simulink model "EF20Algo"  (R2020a)
settings: Solver=VariableStepAuto  StartTime=0.0  StopTime=10.0  RelTol=1e-3
model workspace (MAT data in the model file):
  Batt.init_charge = 100
  Batt.Vnom = 320
  Batt.Ah_rating = 100
  Batt.R1 = 0.0846
  Batt.V1 = 283.3
  Batt.Q1 = 10.4
  Batt.Limit.SOC = [0 10 20 30 40 50 60 70 80 90 100]
  Batt.Limit.Discharge = [0 15000 33000 54000 75000 90000 108000 117000 120000 120000 120000]
  Batt.Limit.Charge = [1 1 1 1 1 1 1 1 0.75 0.35 0]
  Batt.m = 119.7
  Batt.Cp = 101.079756
undefined symbols (not defined in the file): magnitude
libraries: simulink x4
settings Model: Creator=Administrator  LastModifiedBy=Administrator

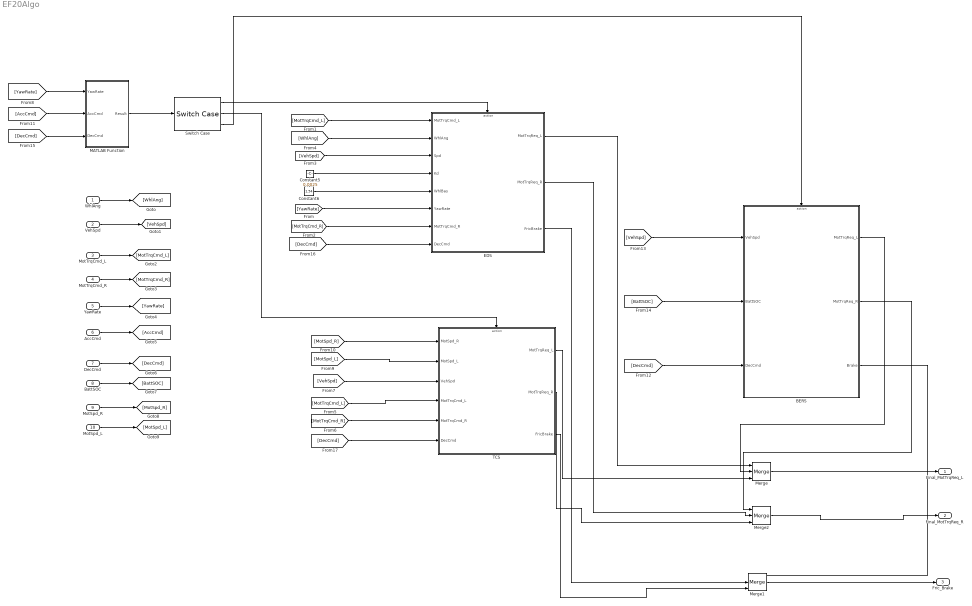
== system EF20Algo ==
  WhlAng : Inport
  VehSpd : Inport  Port=2
  MotTrqCmd_L : Inport  Port=3
  MotTrqCmd_R : Inport  Port=4
  YawRate : Inport  Port=5
  AccCmd : Inport  Port=6
  DecCmd : Inport  Port=7
  BattSOC : Inport  Port=8
  MotSpd_R : Inport  Port=9
  MotSpd_L : Inport  Port=10
  BERS : Subsystem  TreatAsAtomicUnit=on
  Constant5 : Constant  Value=0.0025
  Constant6 : Constant  Value=1.54
  EDS : Subsystem  TreatAsAtomicUnit=on
  MATLAB Function : MATLAB Function  TreatAsAtomicUnit=on
  Merge : Merge  Inputs=3
  Merge1 : Merge  Inputs=3
  Merge2 : Merge  Inputs=3
  Switch Case : SwitchCase  CaseConditions={1,2,3}  ShowDefaultCase=off
  TCS : Subsystem  TreatAsAtomicUnit=on
  Final_MotTrqReq_L : Outport
  Final_MotTrqReq_R : Outport  Port=2
  Fric_Brake : Outport  Port=3
  wires:
  WhlAng/1 -> [WhlAng]
  MotSpd_R/1 -> [MotSpd_R]
  DecCmd/1 -> [DecCmd]
  BattSOC/1 -> [BattSOC]
  MotSpd_L/1 -> [MotSpd_L]
  AccCmd/1 -> [AccCmd]
  YawRate/1 -> [YawRate]
  MotTrqCmd_R/1 -> [MotTrqCmd_R]
  MotTrqCmd_L/1 -> [MotTrqCmd_L]
  VehSpd/1 -> [VehSpd]
  Switch Case/2 -> TCS/Action
  Switch Case/1 -> EDS/Action
  Constant5/1 -> EDS/4(Kd)
  Constant6/1 -> EDS/5(WhlBas)
  [YawRate] -> EDS/6(YawRate)
  [MotTrqCmd_L] -> EDS/1(MotTrqCmd_L)
  [MotTrqCmd_R] -> EDS/7(MotTrqCmd_R)
  [WhlAng] -> EDS/2(WhlAng)
  [VehSpd] -> EDS/3(Spd)
  [MotSpd_L] -> TCS/2(MotSpd_L)
  [MotSpd_R] -> TCS/1(MotSpd_R)
  [VehSpd] -> TCS/3(VehSpd)
  [MotTrqCmd_L] -> TCS/4(MotTrqCmd_L)
  [MotTrqCmd_R] -> TCS/5(MotTrqCmd_R)
  MATLAB Function/1(Result) -> Switch Case/1
  [YawRate] -> MATLAB Function/1(YawRate)
  [AccCmd] -> MATLAB Function/2(AccCmd)
  [VehSpd] -> BERS/1(VehSpd)
  [BattSOC] -> BERS/2(BattSOC)
  [DecCmd] -> BERS/3(DecCmd)
  [DecCmd] -> MATLAB Function/3(DecCmd)
  Switch Case/3 -> BERS/Action
  [DecCmd] -> EDS/8(DecCmd)
  [DecCmd] -> TCS/6(DecCmd)
  Merge1/1 -> Fric_Brake/1
  Merge2/1 -> Final_MotTrqReq_R/1
  Merge/1 -> Final_MotTrqReq_L/1
  EDS/1(MotTrqReq_L) -> Merge/1
  BERS/1(MotTrqReq_L) -> Merge/2
  TCS/1(MotTrqReq_L) -> Merge/3
  BERS/2(MotTrqReq_R) -> Merge2/1
  EDS/2(MotTrqReq_R) -> Merge2/2
  TCS/2(MotTrqReq_R) -> Merge2/3
  BERS/3(Brake) -> Merge1/1
  EDS/3(FricBrake) -> Merge1/2
  TCS/3(FricBrake) -> Merge1/3

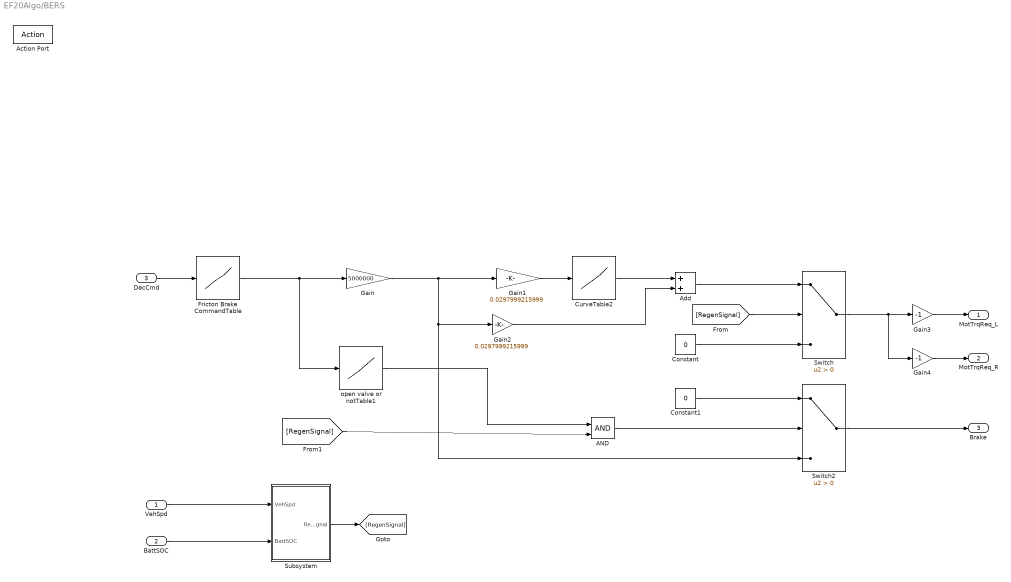
== system EF20Algo/BERS ==
  VehSpd : Inport
  BattSOC : Inport  Port=2
  DecCmd : Inport  Port=3
  Action Port : ActionPort  ActionPortLabel=case [ 3 ]:
  AND : Logic  IconShape=distinctive  AllPortsSameDT=off  OutDataTypeStr=boolean
  Add : Sum
  Constant : Constant  Value=0
  Constant1 : Constant  Value=0
  CurveTable2 : Lookup_n-D  NumberOfTableDimensions=1  BreakpointsForDimension1=Batt.Limit.SOC  Table=Batt.Limit.Charge  InternalRulePriority=Speed  RndMeth=Simplest  InputSameDT=on
  Fricton Brake CommandTable : Lookup_n-D  NumberOfTableDimensions=1  BreakpointsForDimension1=[.0 0.1 0.2 0.4 0.6 0.8 1.0]  Table=[0 0 0.2 0.4 0.6 0.8 1.0]*60  InternalRulePriority=Speed  RndMeth=Simplest  InputSameDT=on
  Gain : Gain  Gain=5000000
  Gain1 : Gain  Gain=0.0297999215999
  Gain2 : Gain  Gain=0.0297999215999
  Gain3 : Gain  Gain=-1
  Gain4 : Gain  Gain=-1
  Subsystem : Subsystem
  Switch : Switch  Criteria=u2 > Threshold
  Switch2 : Switch  Criteria=u2 > Threshold
  open valve or notTable1 : Lookup_n-D  NumberOfTableDimensions=1  BreakpointsForDimension1=[.0 0.1 0.2 0.4 0.6 0.8 1.0]  Table=[0 0 0.2 0.4 0.6 0.8 1.0]*60  InternalRulePriority=Speed  RndMeth=Simplest  InputSameDT=on
  MotTrqReq_L : Outport
  MotTrqReq_R : Outport  Port=2
  Brake : Outport  Port=3
  wires:
  Fricton Brake CommandTable/1 -> open valve or notTable1/1, Gain/1
  Subsystem/1(RegenSignal) -> [RegenSignal]
  Gain3/1 -> MotTrqReq_L/1
  [RegenSignal] -> AND/2
  BattSOC/1 -> Subsystem/2(BattSOC)
  Gain4/1 -> MotTrqReq_R/1
  Gain2/1 -> Add/2
  Switch/1 -> Gain4/1, Gain3/1
  Switch2/1 -> Brake/1
  Gain1/1 -> CurveTable2/1
  CurveTable2/1 -> Add/1
  [RegenSignal] -> Switch/2
  Gain/1 -> Switch2/3, Gain2/1, Gain1/1
  Constant/1 -> Switch/3
  Constant1/1 -> Switch2/1
  VehSpd/1 -> Subsystem/1(VehSpd)
  open valve or notTable1/1 -> AND/1
  Add/1 -> Switch/1
  AND/1 -> Switch2/2
  DecCmd/1 -> Fricton Brake CommandTable/1

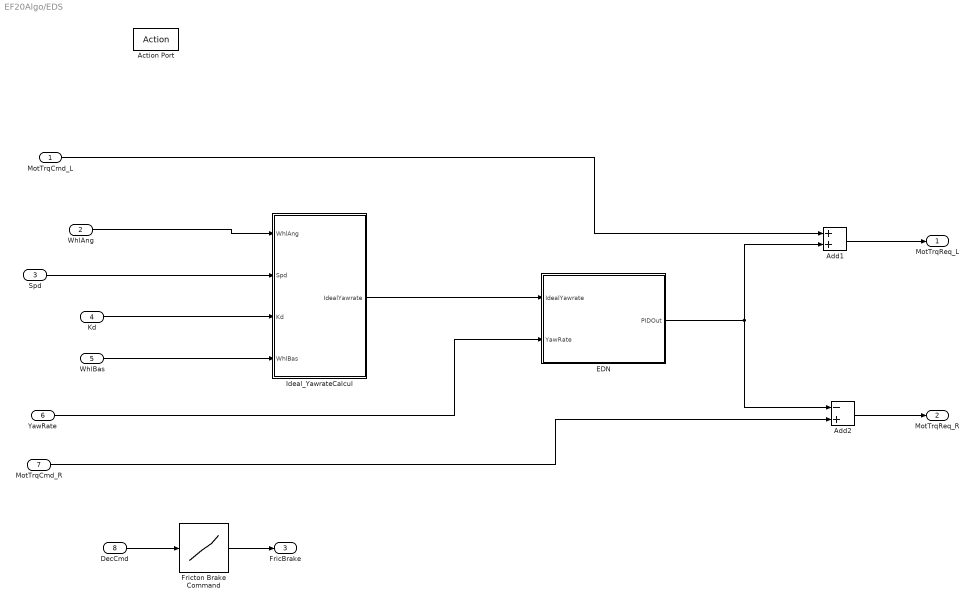
== system EF20Algo/EDS ==
  MotTrqCmd_L : Inport
  WhlAng : Inport  Port=2
  Spd : Inport  Port=3
  Kd : Inport  Port=4
  WhlBas : Inport  Port=5
  YawRate : Inport  Port=6
  MotTrqCmd_R : Inport  Port=7
  DecCmd : Inport  Port=8
  Action Port : ActionPort  ActionPortLabel=case [ 1 ]:
  Add1 : Sum
  Add2 : Sum  Inputs=-+
  EDN : Subsystem
  Fricton Brake Command : Lookup_n-D  NumberOfTableDimensions=1  BreakpointsForDimension1=[.0 0.1 0.2 0.4 0.6 0.8 1.0]  Table=[0 0 0.2 0.4 0.6 0.8 1.0]*60  ExtrapMethod=Clip  InternalRulePriority=Speed  RndMeth=Simplest  InputSameDT=on
  Ideal_YawrateCalcul : Subsystem
  MotTrqReq_L : Outport
  MotTrqReq_R : Outport  Port=2
  FricBrake : Outport  Port=3
  wires:
  Ideal_YawrateCalcul/1(IdealYawrate) -> EDN/1(IdealYawrate)
  Add2/1 -> MotTrqReq_R/1
  Add1/1 -> MotTrqReq_L/1
  YawRate/1 -> EDN/2(YawRate)
  Spd/1 -> Ideal_YawrateCalcul/2(Spd)
  MotTrqCmd_L/1 -> Add1/1
  WhlBas/1 -> Ideal_YawrateCalcul/4(WhlBas)
  Kd/1 -> Ideal_YawrateCalcul/3(Kd)
  WhlAng/1 -> Ideal_YawrateCalcul/1(WhlAng)
  EDN/1(PIDOut) -> Add2/1, Add1/2
  MotTrqCmd_R/1 -> Add2/2
  DecCmd/1 -> Fricton Brake Command/1
  Fricton Brake Command/1 -> FricBrake/1

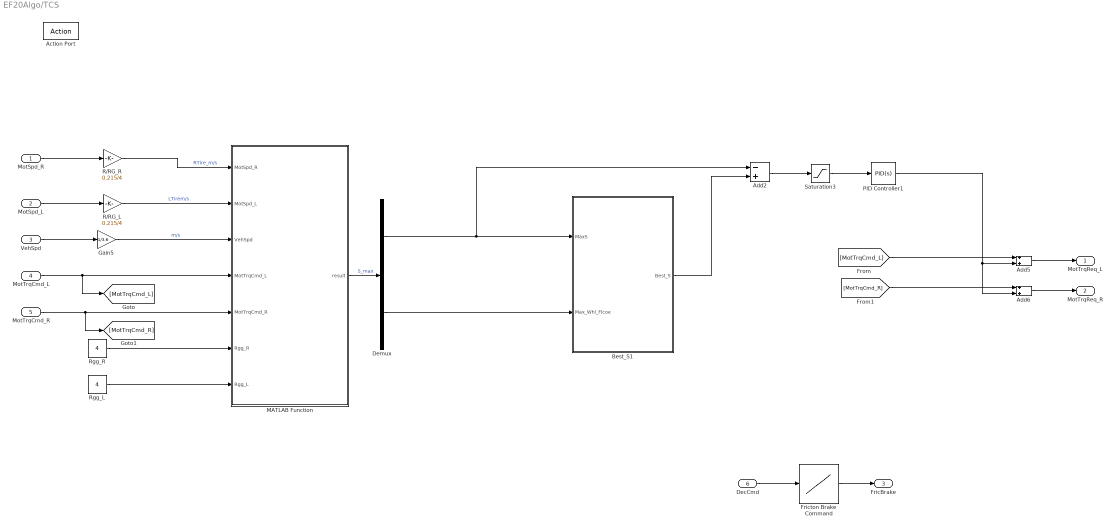
== system EF20Algo/TCS ==
  MotSpd_R : Inport
  MotSpd_L : Inport  Port=2
  VehSpd : Inport  Port=3
  MotTrqCmd_L : Inport  Port=4
  MotTrqCmd_R : Inport  Port=5
  DecCmd : Inport  Port=6
  Action Port : ActionPort  ActionPortLabel=case [ 2 ]:
  Add2 : Sum  Inputs=-+
  Add5 : Sum
  Add6 : Sum
  Best_S1 : Subsystem
  Demux : Demux  Outputs=2
  Fricton Brake Command : Lookup_n-D  NumberOfTableDimensions=1  BreakpointsForDimension1=[.0 0.1 0.2 0.4 0.6 0.8 1.0]  Table=[0 0 0.2 0.4 0.6 0.8 1.0]*60  ExtrapMethod=Clip  InternalRulePriority=Speed  RndMeth=Simplest  InputSameDT=on
  Gain5 : Gain  Gain=1/3.6
  MATLAB Function : MATLAB Function  TreatAsAtomicUnit=on
  PID Controller1 : simulink/Continuous/PID Controller  Controller=PID  Form=Parallel  TimeDomain=Continuous-time  UseExternalTs=off  SampleTime=-1  IntegratorMethod=Forward Euler  FilterMethod=Forward Euler  ControllerParametersSource=internal  P=31  I=1  D=0  UseFilter=on  N=100  TunerSelectOption=Transfer Function Based (PID Tuner App)  InitialConditionSource=internal  InitialConditionForIntegrator=0  InitialConditionForFilter=0  DifferentiatorICPrevScaledInput=0  ExternalReset=none  TrackingMode=off  Kt=1  LimitOutput=off  UpperSaturationLimit=inf  LowerSaturationLimit=-inf  LinearizeAsGain=on  AntiWindupMode=none  Kb=1  POutMin=[]  POutMax=[]  IOutMin=[]  IOutMax=[]  DOutMin=[]  DOutMax=[]  NOutMin=[]  NOutMax=[]  SumOutMin=[]  SumOutMax=[]  SaturationOutMin=[]  SaturationOutMax=[]  PParamMin=[]  PParamMax=[]  IParamMin=[]  IParamMax=[]  DParamMin=[]  DParamMax=[]  NParamMin=[]  NParamMax=[]  KbParamMin=[]  KbParamMax=[]  KtParamMin=[]  KtParamMax=[]  KbOutMin=[]  KbOutMax=[]  KtOutMin=[]  KtOutMax=[]  IntegratorOutMin=[]  IntegratorOutMax=[]  FilterOutMin=[]  FilterOutMax=[]  SumI1OutMin=[]  SumI1OutMax=[]  SumI2OutMin=[]  SumI2OutMax=[]  SumI3OutMin=[]  SumI3OutMax=[]  SumI4OutMin=[]  SumI4OutMax=[]  SumDOutMin=[]  SumDOutMax=[]  DifferentiatorOutMin=[]  DifferentiatorOutMax=[]  FilterDiffOutCoefMin=[]  FilterDiffOutCoefMax=[]  ReciprocalOutMin=[]  ReciprocalOutMax=[]  SumDenOutMin=[]  SumDenOutMax=[]  SumNumOutMin=[]  SumNumOutMax=[]  DivideOutMin=[]  DivideOutMax=[]  UdiffTsProdOutMin=[]  UdiffTsProdOutMax=[]  NTsProdOutMin=[]  NTsProdOutMax=[]  UintegralTsProdOutMin=[]  UintegralTsProdOutMax=[]  UngainTsProdOutMin=[]  UngainTsProdOutMax=[]  IntegratorContinuousStateAttributes=''  IntegratorStateMustResolveToSignalObject=off  IntegratorRTWStateStorageClass=Auto  FilterContinuousStateAttributes=''  FilterStateMustResolveToSignalObject=off  FilterRTWStateStorageClass=Auto  ParallelPVariant=InternalParameters  IdealPVariant=Disabled  IVariant=InternalParameters  DVariant=InternalParameters  IntegratorVariant=Continuous  SatVariant=Disabled  AWVariant=Passthrough  PCopyVariant=Disabled  TRVariant=Disabled  FdbkBlocksVariant=Forward  IdealPFdbkVariant=Disabled  SatFdbkVariant=Disabled  DerivativeFilterVariant=ContFilter  NVariant=InternalParameters  NCopyVariant=Disabled  FilterICVariant=InternalICsFilter  IntegratorICVariant=InternalICs  ExternalResetVariant=Disabled  TRSumVariant=Passthrough  SumFdbkVariant=Disabled  SumVariant=Sum_PID  TsampFilterVariant=InternalTs  TsampNgainVariant=Passthrough  TsampIntegralVariant=Passthrough
  R/RG_L : Gain  Gain=0.215/4
  R/RG_R : Gain  Gain=0.215/4
  Rgg_L : Constant  Value=4
  Rgg_R : Constant  Value=4
  Saturation3 : Saturate  UpperLimit=2  LowerLimit=-2
  MotTrqReq_L : Outport
  MotTrqReq_R : Outport  Port=2
  FricBrake : Outport  Port=3
  wires:
  [MotTrqCmd_R] -> Add6/1
  Add5/1 -> MotTrqReq_L/1
  Gain5/1 -> MATLAB Function/3(VehSpd)  "m/s"
  MotTrqCmd_R/1 -> [MotTrqCmd_R], MATLAB Function/5(MotTrqCmd_R)
  R/RG_L/1 -> MATLAB Function/2(MotSpd_L)  "LTirem/s"
  R/RG_R/1 -> MATLAB Function/1(MotSpd_R)  "RTire_m/s"
  Saturation3/1 -> PID Controller1/1
  PID Controller1/1 -> Add6/2, Add5/2
  [MotTrqCmd_L] -> Add5/1
  Add6/1 -> MotTrqReq_R/1
  MotTrqCmd_L/1 -> [MotTrqCmd_L], MATLAB Function/4(MotTrqCmd_L)
  MotSpd_L/1 -> R/RG_L/1
  VehSpd/1 -> Gain5/1
  Rgg_R/1 -> MATLAB Function/6(Rgg_R)
  MotSpd_R/1 -> R/RG_R/1
  Best_S1/1(Best_S) -> Add2/2
  Add2/1 -> Saturation3/1
  Rgg_L/1 -> MATLAB Function/7(Rgg_L)
  DecCmd/1 -> Fricton Brake Command/1
  Fricton Brake Command/1 -> FricBrake/1
  MATLAB Function/1(result) -> Demux/1  "S_max"
  Demux/1 -> Add2/1, Best_S1/1(MaxS)
  Demux/2 -> Best_S1/2(Max_Whl_Flcoe)

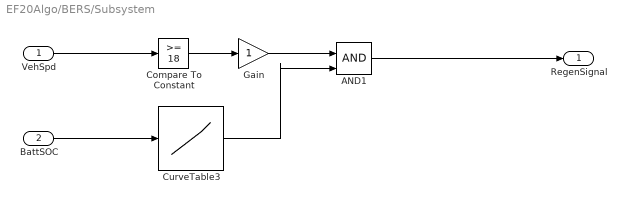
== system EF20Algo/BERS/Subsystem ==
  VehSpd : Inport
  BattSOC : Inport  Port=2
  AND1 : Logic  IconShape=distinctive  AllPortsSameDT=off  OutDataTypeStr=boolean
  Compare To Constant : simulink/Logic and Bit Operations/Compare To Constant  relop=>=  const=18  OutDataTypeStr=boolean
  CurveTable3 : Lookup_n-D  NumberOfTableDimensions=1  BreakpointsForDimension1=Batt.Limit.SOC  BreakpointsForDimension1DataTypeStr=Inherit: Inherit from 'Breakpoint data'  Table=Batt.Limit.Charge  ExtrapMethod=Clip  UseLastTableValue=on  InternalRulePriority=Speed  RndMeth=Simplest  InputSameDT=on
  Gain : Gain
  RegenSignal : Outport
  wires:
  VehSpd/1 -> Compare To Constant/1
  CurveTable3/1 -> AND1/2
  BattSOC/1 -> CurveTable3/1
  AND1/1 -> RegenSignal/1
  Gain/1 -> AND1/1
  Compare To Constant/1 -> Gain/1

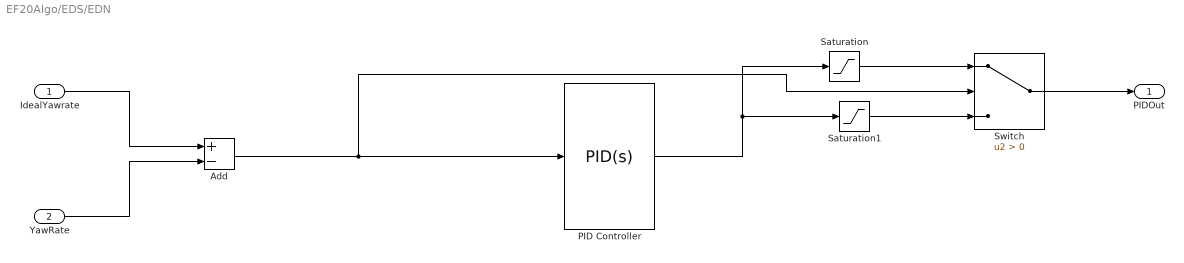
== system EF20Algo/EDS/EDN ==
  IdealYawrate : Inport
  YawRate : Inport  Port=2
  Add : Sum  Inputs=+-
  PID Controller : simulink/Continuous/PID Controller  Controller=PID  Form=Parallel  TimeDomain=Continuous-time  UseExternalTs=off  SampleTime=-1  IntegratorMethod=Forward Euler  FilterMethod=Forward Euler  ControllerParametersSource=internal  P=2  I=1  D=0  UseFilter=on  N=100  TunerSelectOption=Transfer Function Based (PID Tuner App)  InitialConditionSource=internal  InitialConditionForIntegrator=0  InitialConditionForFilter=0  DifferentiatorICPrevScaledInput=0  ExternalReset=none  TrackingMode=off  Kt=1  LimitOutput=on  UpperSaturationLimit=30  LowerSaturationLimit=-30  LinearizeAsGain=on  AntiWindupMode=none  Kb=1  SaturateOnIntegerOverflow=on  POutMin=[]  POutMax=[]  IOutMin=[]  IOutMax=[]  DOutMin=[]  DOutMax=[]  NOutMin=[]  NOutMax=[]  SumOutMin=[]  SumOutMax=[]  SaturationOutMin=[]  SaturationOutMax=[]  PParamMin=[]  PParamMax=[]  IParamMin=[]  IParamMax=[]  DParamMin=[]  DParamMax=[]  NParamMin=[]  NParamMax=[]  KbParamMin=[]  KbParamMax=[]  KtParamMin=[]  KtParamMax=[]  KbOutMin=[]  KbOutMax=[]  KtOutMin=[]  KtOutMax=[]  IntegratorOutMin=[]  IntegratorOutMax=[]  FilterOutMin=[]  FilterOutMax=[]  SumI1OutMin=[]  SumI1OutMax=[]  SumI2OutMin=[]  SumI2OutMax=[]  SumI3OutMin=[]  SumI3OutMax=[]  SumI4OutMin=[]  SumI4OutMax=[]  SumDOutMin=[]  SumDOutMax=[]  DifferentiatorOutMin=[]  DifferentiatorOutMax=[]  FilterDiffOutCoefMin=[]  FilterDiffOutCoefMax=[]  ReciprocalOutMin=[]  ReciprocalOutMax=[]  SumDenOutMin=[]  SumDenOutMax=[]  SumNumOutMin=[]  SumNumOutMax=[]  DivideOutMin=[]  DivideOutMax=[]  UdiffTsProdOutMin=[]  UdiffTsProdOutMax=[]  NTsProdOutMin=[]  NTsProdOutMax=[]  UintegralTsProdOutMin=[]  UintegralTsProdOutMax=[]  UngainTsProdOutMin=[]  UngainTsProdOutMax=[]  IntegratorContinuousStateAttributes=''  IntegratorStateMustResolveToSignalObject=off  IntegratorRTWStateStorageClass=Auto  FilterContinuousStateAttributes=''  FilterStateMustResolveToSignalObject=off  FilterRTWStateStorageClass=Auto  ParallelPVariant=InternalParameters  IdealPVariant=Disabled  IVariant=InternalParameters  DVariant=InternalParameters  IntegratorVariant=Continuous  SatVariant=Enabled  AWVariant=Passthrough  PCopyVariant=Disabled  TRVariant=Disabled  FdbkBlocksVariant=Forward  IdealPFdbkVariant=Disabled  SatFdbkVariant=Disabled  DerivativeFilterVariant=ContFilter  NVariant=InternalParameters  NCopyVariant=Disabled  FilterICVariant=InternalICsFilter  IntegratorICVariant=InternalICs  ExternalResetVariant=Disabled  TRSumVariant=Passthrough  SumFdbkVariant=Disabled  SumVariant=Sum_PID  TsampFilterVariant=InternalTs  TsampNgainVariant=Passthrough  TsampIntegralVariant=Passthrough
  Saturation : Saturate  UpperLimit=inf  LowerLimit=0
  Saturation1 : Saturate  UpperLimit=0  LowerLimit=-inf
  Switch : Switch  Criteria=u2 > Threshold
  PIDOut : Outport
  wires:
  Add/1 -> Switch/2, PID Controller/1
  Saturation/1 -> Switch/1
  Switch/1 -> PIDOut/1
  Saturation1/1 -> Switch/3
  YawRate/1 -> Add/2
  IdealYawrate/1 -> Add/1
  PID Controller/1 -> Saturation1/1, Saturation/1

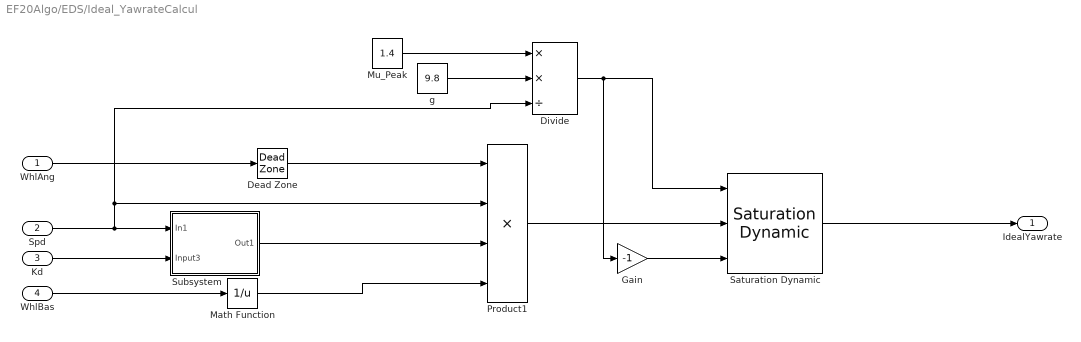
== system EF20Algo/EDS/Ideal_YawrateCalcul ==
  WhlAng : Inport
  Spd : Inport  Port=2
  Kd : Inport  Port=3
  WhlBas : Inport  Port=4
  Dead Zone : DeadZone  LowerValue=-0.025  UpperValue=0.025  SaturateOnIntegerOverflow=on
  Divide : Product  Inputs=**/
  Gain : Gain  Gain=-1
  Math Function : Math  Operator=reciprocal  SaturateOnIntegerOverflow=on
  Mu_Peak : Constant  Value=1.4
  Product1 : Product  Inputs=4
  Saturation Dynamic : simulink/Discontinuities/Saturation Dynamic  OutMin=[]  OutMax=[]  OutDataTypeStr=Inherit: Same as second input  OutDataType=fixdt(1, 16)  OutScaling=2^-10  DoSatur=off
  Subsystem : Subsystem
  g : Constant  Value=9.8
  IdealYawrate : Outport
  wires:
  Spd/1 -> Divide/3, Product1/2, Subsystem/1(In1)
  Product1/1 -> Saturation Dynamic/2
  Divide/1 -> Gain/1, Saturation Dynamic/1
  g/1 -> Divide/2
  Mu_Peak/1 -> Divide/1
  Subsystem/1(Out1) -> Product1/3
  WhlAng/1 -> Dead Zone/1
  Saturation Dynamic/1 -> IdealYawrate/1
  Gain/1 -> Saturation Dynamic/3
  WhlBas/1 -> Math Function/1
  Kd/1 -> Subsystem/2(Input3)
  Math Function/1 -> Product1/4
  Dead Zone/1 -> Product1/1

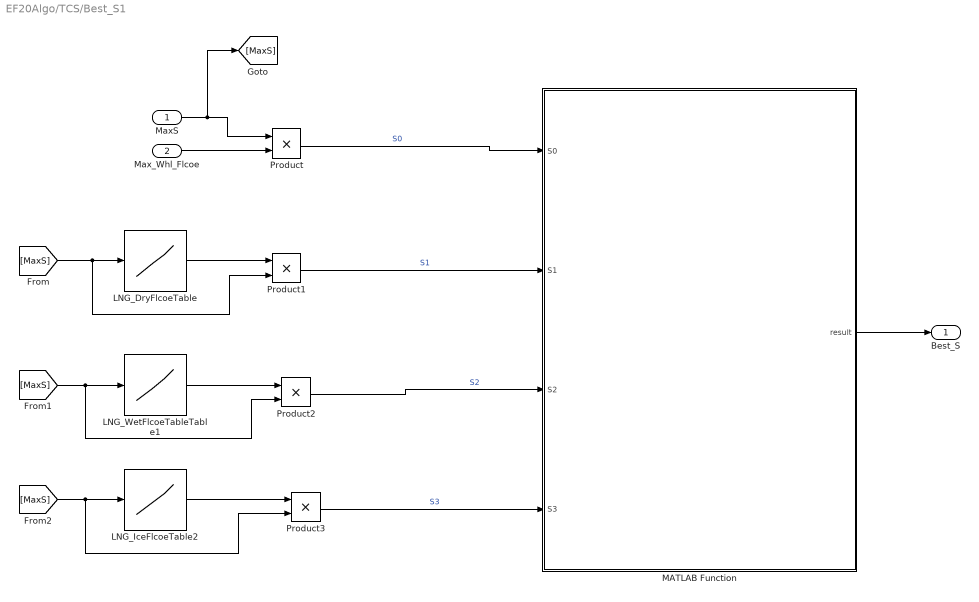
== system EF20Algo/TCS/Best_S1 ==
  MaxS : Inport
  Max_Whl_Flcoe : Inport  Port=2
  LNG_DryFlcoeTable : Lookup_n-D  NumberOfTableDimensions=1  BreakpointsForDimension1="[0\t0.02\t0.04\t0.06\t0.08\t0.1\t0.12\t0.14\t0.16\t0.18\t0.2\t0.22\t0.24\t0.26\t0.28\t0.3\t0.32\t0.34\t0.36\t0.38\t0.4\t0.42\t0.44\t0.46\t0.48\t0.5\t0.52\t0.54\t0.56\t0.58\t0.6\t0.62\t0.64\t0.66\t0.68\t0.7\t0.72\t0.74\t0.76\t0.78\t0.8\t0.82\t0.84\t0.86\t0.88\t0.9\t0.92\t0.94\t0.96\t0.98\t1]"  Table="[0\t0.463\t0.738\t0.9\t0.994\t1.05\t1.07\t1.09\t1.09\t1.09\t1.08\t1.07\t1.06\t1.05\t1.04\t1.03\t1.02\t1.01\t1\t0.992\t0.981\t0.97\t0.959\t0.949\t0.938\t0.927\t0.916\t0.905\t0.895\t0.884\t0.873\t0.862\t0.851\t0.841\t0.83\t0.819\t0.808\t0.797\t0.787\t0.776\t0.765\t0.754\t0.743\t0.733\t0.722\t0.711\t0.7\t0.689\t0.679\t0.668\t0.657]"  InternalRulePriority=Speed  RndMeth=Simplest  InputSameDT=on
  LNG_IceFlcoeTable2 : Lookup_n-D  NumberOfTableDimensions=1  BreakpointsForDimension1=[ 0, 0.02, 0.04, 0.06, 0.08, 0.1, 0.12, 0.14, 0.16, 0.18, 0.2, 0.22, 0.24, 0.26, 0.28, 0.3, 0.32, 0.34, 0.36, 0.38, 0.4, 0.42, 0.44, 0.46, 0.48, 0.5, 0.52, 0.54, 0.56, 0.58, 0.6, 0.62, 0.64, 0.66, 0.68, 0.7, 0.72, 0.74, 0.76, 0.78, 0.8, 0.82, 0.84, 0.86, 0.88, 0.9, 0.92, 0.94, 0.96, 0.98, 1.0]  Table=[ 0, 0.05, 0.05, 0.05, 0.05, 0.05, 0.05, 0.05, 0.05, 0.05, 0.05, 0.05, 0.05, 0.05, 0.05, 0.05, 0.05, 0.05, 0.05, 0.05, 0.05, 0.05, 0.05, 0.05, 0.05, 0.05, 0.05, 0.05, 0.049, 0.049, 0.049, 0.049, 0.049, 0.049, 0.049, 0.049, 0.049, 0.049, 0.049, 0.049, 0.049, 0.049, 0.049, 0.049, 0.049, 0.049, 0.049, 0.049, 0.049, 0.049, 0.049]  InternalRulePriority=Speed  RndMeth=Simplest  InputSameDT=on
  LNG_WetFlcoeTableTable1 : Lookup_n-D  NumberOfTableDimensions=1  BreakpointsForDimension1=[ 0, 0.02, 0.04, 0.06, 0.08, 0.1, 0.12, 0.14, 0.16, 0.18, 0.2, 0.22, 0.24, 0.26, 0.28, 0.3, 0.32, 0.34, 0.36, 0.38, 0.4, 0.42, 0.44, 0.46, 0.48, 0.5, 0.52, 0.54, 0.56, 0.58, 0.6, 0.62, 0.64, 0.66, 0.68, 0.7, 0.72, 0.74, 0.76, 0.78, 0.8, 0.82, 0.84, 0.86, 0.88, 0.9, 0.92, 0.94, 0.96, 0.98, 1.0]  Table=[ 0, 0.41, 0.62, 0.72, 0.77, 0.79, 0.8, 0.8, 0.8, 0.79, 0.79, 0.78, 0.77, 0.77, 0.76, 0.75, 0.74, 0.74, 0.73, 0.72, 0.72, 0.71, 0.7, 0.7, 0.69, 0.68, 0.68, 0.67, 0.66, 0.65, 0.65, 0.64, 0.63, 0.63, 0.62, 0.61, 0.6, 0.6, 0.59, 0.58, 0.58, 0.57, 0.56, 0.56, 0.55, 0.54, 0.54, 0.53, 0.52, 0.51, 0.51]  InternalRulePriority=Speed  RndMeth=Simplest  InputSameDT=on
  MATLAB Function : MATLAB Function  TreatAsAtomicUnit=on
  Product{,1..3} (4 alike) : Product
  Best_S : Outport
  wires:
  Product3/1 -> MATLAB Function/4(S3)  "S3"
  Product2/1 -> MATLAB Function/3(S2)  "S2"
  Product1/1 -> MATLAB Function/2(S1)  "S1"
  Product/1 -> MATLAB Function/1(S0)  "S0"
  LNG_IceFlcoeTable2/1 -> Product3/1
  LNG_WetFlcoeTableTable1/1 -> Product2/1
  LNG_DryFlcoeTable/1 -> Product1/1
  [MaxS] -> LNG_WetFlcoeTableTable1/1, Product2/2
  [MaxS] -> LNG_IceFlcoeTable2/1, Product3/2
  [MaxS] -> LNG_DryFlcoeTable/1, Product1/2
  Max_Whl_Flcoe/1 -> Product/2
  MaxS/1 -> Product/1, [MaxS]
  MATLAB Function/1(result) -> Best_S/1

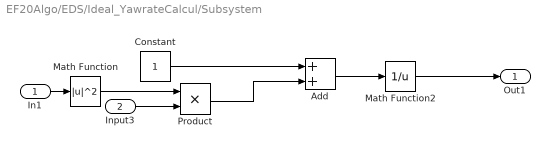
== system EF20Algo/EDS/Ideal_YawrateCalcul/Subsystem ==
  In1 : Inport
  Input3 : Inport  Port=2
  Add : Sum
  Constant : Constant
  Math Function : Math  Operator=magnitude^2  SaturateOnIntegerOverflow=on
  Math Function2 : Math  Operator=reciprocal  SaturateOnIntegerOverflow=on
  Product : Product
  Out1 : Outport
  wires:
  Add/1 -> Math Function2/1
  Product/1 -> Add/2
  Input3/1 -> Product/2
  Math Function2/1 -> Out1/1
  Math Function/1 -> Product/1
  Constant/1 -> Add/1
  In1/1 -> Math Function/1

== matlab function EF20Algo/MATLAB Function ==
  data: YawRate input; Result output double size=1; AccCmd input; DecCmd input
function Result = fcn(YawRate,AccCmd,DecCmd)
if abs(YawRate)<0.025&&AccCmd>0
    out = 2;
elseif DecCmd>0
    out = 3;
else
    out = 1;
end

Result = out;
end

== matlab function EF20Algo/TCS/MATLAB Function ==
  data: MotSpd_R input; result output double size=2; MotSpd_L input; VehSpd input; MotTrqCmd_L input; MotTrqCmd_R input; Rgg_R input; Rgg_L input
function result = fcn(MotSpd_R,MotSpd_L,VehSpd,MotTrqCmd_L,MotTrqCmd_R,Rgg_R,Rgg_L)
S_r = (MotSpd_R - VehSpd)/MotSpd_R;
S_l = (MotSpd_L - VehSpd)/MotSpd_L;
 if(S_r>S_l)
     S_max = S_r;
     u_max = (MotTrqCmd_R*Rgg_R*0.95)/0.215/(330*0.55*0.5);
 else
     S_max = S_l;
     u_max = (MotTrqCmd_L*Rgg_L*0.95)/0.215/(330*0.55*0.5);
 end
result = [S_max;u_max];
end

== matlab function EF20Algo/TCS/Best_S1/MATLAB Function ==
  data: S0 input; result output; S1 input; S2 input; S3 input
function result = fcn(S0,S1,S2,S3)
    a = abs(S0-S1);a1=0.16;
    b=abs(S0-S2);b1=0.131;
    c = abs(S0-S3);c1=0.031;
    if a>b
        if b>c
            best_S = c1;
        else
            best_S =b1;
        end
    else
       if a>c
           best_S = c1;
       else
           best_S = a1;
       end
    end
result = best_S;
end
